simulink model "OFDM"  (R2016b)
settings: Solver=FixedStepDiscrete  StartTime=0.0  StopTime=10.0  RelTol=1e-3
libraries: commdigbbndam3 x16, hdlsllib x2
settings Model: DataTypeOverride=Off  Creator=jake  LastModifiedBy=jake
settings DataIOCC: SaveOutput=off  SaveTime=off
settings OptimizationCC: BlockReduction=off  ConditionallyExecuteInputs=off  DefaultParameterBehavior=Inlined
settings DebuggingCC: AlgebraicLoopMsg=error  SingleTaskRateTransMsg=error  StrictBusMsg=ErrorOnBusTreatedAsVector
settings HardwareCC: ProdBitPerPointer=32  ProdBitPerSizeT=32  ProdBitPerPtrDiffT=32  ProdLargestAtomicFloat=None  ProdIntDivRoundTo=Undefined  ProdEndianess=Unspecified  ProdWordSize=32  ProdHWDeviceType=ASIC/FPGA->ASIC/FPGA  ProdEqTarget=off
settings GRTTargetCC: TargetLangStandard=C89/C90 (ANSI)

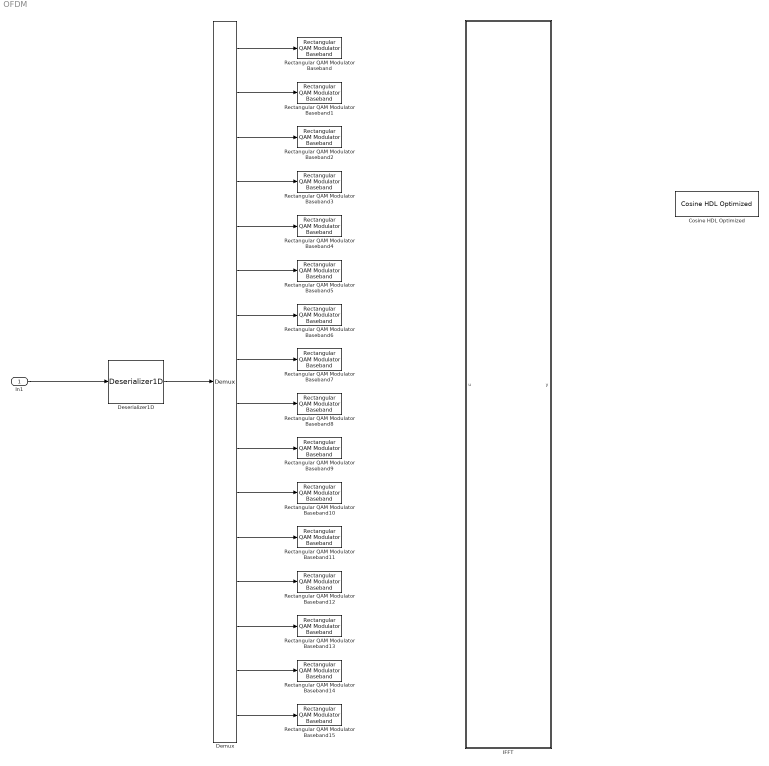
== system OFDM ==
  In1 : Inport
  Cosine HDL Optimized : hdlsllib/Lookup Tables/Cosine HDL Optimized  OutputFormula=cos(2*pi*u)  NumDataPoints=64  TableDataTypeStr=fixdt(0,16,15)  SimulateLUTROMDelay=off
  Demux : Demux  Outputs=16  BusSelectionMode=on
  Deserializer1D : hdlsllib/HDL Operations/Deserializer1D  Ratio=8  IdleCycles=0  InitialCondition=0  startIn=off  validIn=off  validOut=off  inputDataDimensions=-1  inputSampleTime=-1  inputSignalType=auto
  IFFT : MATLAB Function  TreatAsAtomicUnit=on
  Rectangular QAM Modulator Baseband{,1..15} (16 alike) : commdigbbndam3/Rectangular QAM Modulator Baseband  M=16  InType=Integer  Enc=Gray  Mapping=[0:15]  PowType=Min. distance between symbols  MinDist=2  AvgPow=1  PeakPow=1  Ph=0  outDtype=double  outWordLen=16  outUDDataType=sfix(16)  outFracLenMode=Best precision  outFracLen=15  outDataTypeStr=double  outLastDataTypeStr=double
  wires:
  In1/1 -> Deserializer1D/1
  Demux/1 -> Rectangular QAM Modulator Baseband/1
  Demux/2 -> Rectangular QAM Modulator Baseband1/1
  Demux/3 -> Rectangular QAM Modulator Baseband2/1
  Demux/4 -> Rectangular QAM Modulator Baseband3/1
  Demux/5 -> Rectangular QAM Modulator Baseband4/1
  Deserializer1D/1 -> Demux/1
  Demux/6 -> Rectangular QAM Modulator Baseband5/1
  Demux/7 -> Rectangular QAM Modulator Baseband6/1
  Demux/8 -> Rectangular QAM Modulator Baseband7/1
  Demux/9 -> Rectangular QAM Modulator Baseband8/1
  Demux/10 -> Rectangular QAM Modulator Baseband9/1
  Demux/11 -> Rectangular QAM Modulator Baseband10/1
  Demux/12 -> Rectangular QAM Modulator Baseband11/1
  Demux/13 -> Rectangular QAM Modulator Baseband12/1
  Demux/14 -> Rectangular QAM Modulator Baseband13/1
  Demux/15 -> Rectangular QAM Modulator Baseband14/1
  Demux/16 -> Rectangular QAM Modulator Baseband15/1

== matlab function OFDM/IFFT ==
  data: u input; y output
function y = fcn(u)
%#codegen

y = u;
